simulink model "hware_long"  (R2012b)
settings: Solver=ode45  StartTime=0.0  StopTime=1500  RelTol=1e-3
libraries: xbsIndex_r4 x265, xps_library x7, casper_library_misc x2, casper_library_delays x2, casper_library_reorder x1
(part 2 of 4)

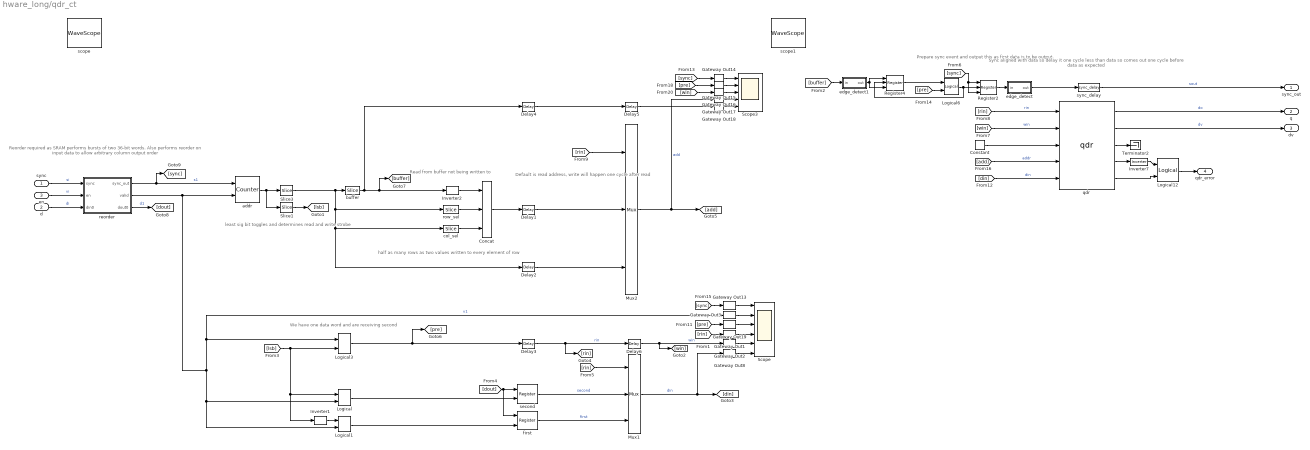
== system hware_long/qdr_ct ==
  note: Reorder required as SRAM performs
      | bursts of two 36-bit words.
      | Also performs reorder on input
      | data to allow arbitrary column
      | output order
  note: Prepare sync event and output
      | this as first data is to be output.
  note: Sync aligned with data so
      | delay it one cycle less
      | than data so comes out one
      | cycle before data as
      | expected
  note: least sig bit toggles
      | and determines read
      | and write strobe
  note: We have one data word
      | and are receiving second
  note: Default is read address,
      | write will happen one
      | cycle after read
  note: Read from buffer
      | not being
      | written to
  note: half as many rows
      | as two values
      | written to every
      | element of row
  sync : Inport
  d : Inport  Port=2
  en : Inport  Port=3
  Concat : xbsIndex_r4/Concat  num_inputs=3  dbl_ovrd=off  block_type=concat
      settings: block_version=10.1.3
  Constant : xbsIndex_r4/Constant  const=15  gui_display_data_type=Fixed-point  arith_type=Unsigned  n_bits=4  bin_pt=0  preci_type=Single  exp_width=8  frac_width=24  explicit_period=on  period=1  equ=P=C  opselect=C  inp2=PCIN>>17  opr=+  inp1=P  carry=CIN  dbl_ovrd=off  block_type=constant
  Delay{1..6} (6 alike) : xbsIndex_r4/Delay  rst=off  infoeditControl=Selection of Reset will increase slice count due to use of real FFs and instead of SRLs  en=off  latency=1  dbl_ovrd=off  reg_retiming=off  block_type=delay
      settings: block_version=11.4
  Gateway Out{1..3,8,13..19} (11 alike) : xbsIndex_r4/Gateway Out  inherit_from_input=off  hdl_port=off  timing_constraint=None  locs_specified=off  LOCs={}  UseAsDAC=off  DACChannel='1'  block_type=gatewayout
      settings: infoedit="Gateway out block.  Converts Xilinx fixed point inputs into ouputs of type Simulink integer, double, or fixed point.<br><br>Hardware notes:  In hardware these blocks become top level output ports or are discarded, depending on how they are configured."  block_version=11.4
  Inverter1 : xbsIndex_r4/Inverter  en=off  latency=0  dbl_ovrd=off  block_type=inv
  Inverter2 : xbsIndex_r4/Inverter  en=off  latency=0  dbl_ovrd=off  block_type=inv
  Inverter7 : xbsIndex_r4/Inverter  en=off  latency=0  dbl_ovrd=off  block_type=inv
      settings: block_version=11.4
  Logical{,1,3,6} (4 alike) : xbsIndex_r4/Logical  logical_function=AND  inputs=2  en=off  latency=0  precision=Full  arith_type=Unsigned  n_bits=16  bin_pt=0  align_bp=on  dbl_ovrd=off  block_type=logical
      settings: block_version=11.4
  Logical12 : xbsIndex_r4/Logical  logical_function=OR  inputs=2  en=off  latency=1  precision=Full  arith_type=Unsigned  n_bits=8  bin_pt=2  align_bp=on  dbl_ovrd=off  block_type=logical
      settings: xl_area=[0, 0, 0, 0, 0, 0, 0]
  Mux1 : xbsIndex_r4/Mux  inputs=2  en=off  latency=1  precision=Full  arith_type=Unsigned  n_bits=16  bin_pt=14  quantization=Truncate  overflow=Wrap  dbl_ovrd=off  block_type=mux
      settings: block_version=11.4
  Mux2 : xbsIndex_r4/Mux  inputs=2  en=off  latency=1  precision=Full  arith_type=Unsigned  n_bits=16  bin_pt=14  quantization=Truncate  overflow=Wrap  dbl_ovrd=off  block_type=mux
      settings: block_version=11.4
  Register2 : xbsIndex_r4/Register  init=0  rst=on  en=on  dbl_ovrd=off  block_type=register
      settings: block_version=11.4
  Register4 : xbsIndex_r4/Register  init=0  rst=on  en=on  dbl_ovrd=off  block_type=register
      settings: block_version=11.4
  Scope : Scope  NumInputPorts=6
      settings: YMin=0~0~0~0~0~0  YMax=1~1~1~1~1~15
  Scope3 : Scope  NumInputPorts=5
      settings: TimeRange=27.56125882301808  YMin=0~0~0~0~0  YMax=1~1~600~15~1  SaveName=ScopeData4
  Slice1 : xbsIndex_r4/Slice  nbits=1  boolean_output=on  mode=Lower Bit Location + Width  bit1=0  base1=MSB of Input  bit0=0  base0=LSB of Input  dbl_ovrd=off  block_type=slice
      settings: block_version=10.1.3
  Slice3 : xbsIndex_r4/Slice  nbits=(idepth + odepth + 1) - 1  boolean_output=off  mode=Upper Bit Location + Width  bit1=0  base1=MSB of Input  bit0=0  base0=LSB of Input  dbl_ovrd=off  block_type=slice
      settings: block_version=10.1.3
  Terminator2 : Terminator
  addr : xbsIndex_r4/Counter  cnt_type=Free Running  cnt_to=Inf  operation=Up  start_count=0  cnt_by_val=1  arith_type=Unsigned  n_bits=(idepth + odepth + 1)  bin_pt=0  load_pin=off  rst=on  en=on  explicit_period=on  period=1  dbl_ovrd=off  use_behavioral_HDL=off  implementation=Fabric  use_rpm=off  block_type=counter
  buffer : xbsIndex_r4/Slice  nbits=1  boolean_output=on  mode=Upper Bit Location + Width  bit1=0  base1=MSB of Input  bit0=0  base0=LSB of Input  dbl_ovrd=off  block_type=slice
      settings: block_version=10.1.3
  col_sel : xbsIndex_r4/Slice  nbits=idepth  boolean_output=off  mode=Lower Bit Location + Width  bit1=0  base1=MSB of Input  bit0=odepth-1  base0=LSB of Input  dbl_ovrd=off  block_type=slice
      settings: block_version=10.1.3
  edge_detect : Subsystem  AncestorBlock=casper_library_misc/edge_detect  mask(edge_detect){edge=Falling, polarity=Active High, x_in=[0 0.08 0.08 0.16 0.16 0.24 0.24 0.32 0.32 0.4], y_in=[1  1 -1 -1 -1 -1 -1 -1 -1 -1], x_out=[0.6 0.68 0.68 0.76 0.76 0.84 0.84 0.92 0.92 1], y_out=[-1 -1  1  1 -1 -1 -1 -1 -1 -1]}
      mask prompts: edge "Edge Type"; polarity "Output Polarity"; x_in "Input X Positions"; y_in "Input Y Positions"; x_out "Output X Positions"; y_out "Output Y Positions"
      mask help: Output is active for one-cycle after each edge of the specified type (i.e. rising, falling or both).
      mask init:
      | edge_detect_init(gcb,...
      |     'edge',edge,...
      |     'polarity',polarity,...
      |     'x_in',x_in,...
      |     'x_out',x_out,...
      |     'y_in',y_in,...
      |     'y_out',y_out);
      | 
      | x_in_num=str2num(getfield(getfield(get_param(gcb,'UserData'),'parameters'),'x_in'));
      | x_out_num=str2num(getfield(getfield(get_param(gcb,'UserData'),'parameters'),'x_out'));
      | y_in_num=str2num(getfield(getfield(get_param(gcb,'UserData'),'parameters'),'y_in'));
      | y_out_num=str2num(getfield(getfield(get_param(gcb,'UserData'),'parameters'),'y_out'));
      settings: AttributesFormatString=|
      | falling edges
      | active high
      mask Help: Output is active for one-cycle after each edge of the specified type (i.e. rising, falling, or both).  Latency is zero.
      mask TypeOptions edge: Rising | Falling | Both
      mask TypeOptions polarity: Active High | Active Low
      mask Display:
      | plot(x_in_num,0.5+y_in_num*0.2);
      | plot(x_out_num,0.5+y_out_num*0.2);
  edge_detect1 : Subsystem  AncestorBlock=casper_library_misc/edge_detect  mask(edge_detect){edge=Rising, polarity=Active High, x_in=[0 0.08 0.08 0.16 0.16 0.24 0.24 0.32 0.32 0.4], y_in=[-1 -1  1  1  1  1  1  1  1  1], x_out=[0.6 0.68 0.68 0.76 0.76 0.84 0.84 0.92 0.92 1], y_out=[-1 -1  1  1 -1 -1 -1 -1 -1 -1]}
      mask prompts: edge "Edge Type"; polarity "Output Polarity"; x_in "Input X Positions"; y_in "Input Y Positions"; x_out "Output X Positions"; y_out "Output Y Positions"
      mask help: Output is active for one-cycle after each edge of the specified type (i.e. rising, falling or both).
      mask init: same as hware_long/qdr_ct/edge_detect
      settings: AttributesFormatString=|
      | rising edges
      | active high
      mask Help: Output is active for one-cycle after each edge of the specified type (i.e. rising, falling, or both).  Latency is zero.
      mask TypeOptions edge: Rising | Falling | Both
      mask TypeOptions polarity: Active High | Active Low
      mask Display:
      | plot(x_in_num,0.5+y_in_num*0.2);
      | plot(x_out_num,0.5+y_out_num*0.2);
  first : xbsIndex_r4/Register  init=0  rst=off  en=on  dbl_ovrd=off  block_type=register
      settings: block_version=11.4
  qdr : xps_library/qdr  Tag=xps:qdr  which_qdr=qdr0  qdr_awidth=20  use_sniffer=off
  reorder : Subsystem  AncestorBlock=casper_library_reorder/reorder  mask(reorder){map=[0   65536       1   65537       2   65538       3   65539       4   65540       5   65541       6   65542       7   65543       8   65544       9   65545      10   65546      11   65547      12   65548      13   65549      14   65550      15   65551      16   65552      17   65553      18   65554      19   65555      20   65556      21   65557      22   65558      23   65559      24   65560      25   65561      26   65562      27   65563      28   65564      29   65565      30   65566      31   65567      32   65568      33   65569      34   65570      35   65571      36   65572      37   65573      38   65574      39   65575      40   65576      41   65577      42   65578      43   65579      44   65580      45   65581      46   65582      47   65583      48   65584      49   65585      50   65586      51   65587      52   65588      53   65589      54   65590      55   65591      56   65592      57   65593      58   65594      59   65595      60   65596      61   65597      62   65598      63   65599      64   65600      65   65601      66   65602      67   65603      68   65604      69   65605      70   65606      71   65607      72   65608      73   65609      74   65610      75   65611      76   65612      77   65613      78   65614      79   65615      80   65616      81   65617      82   65618      83   65619      84   65620      85   65621      86   65622      87   65623      88   65624      89   65625      90   65626      91   65627      92   65628      93   65629      94   65630      95   65631      96   65632      97   65633      98   65634      99   65635     100   65636     101   65637     102   65638     103   65639     104   65640     105   65641     106   65642     107   65643     108   65644     109   65645     110   65646     111   65647     112   65648     113   65649     114   65650     115   65651     116   65652     117   65653     118   65654     119   65655     120   65656     121   65657     122   65658     123   65659     124   65660     125   65661     126   65662     127   65663     128   65664     129   65665     130   65666     131   65667     132   65668     133   65669     134   65670     135   65671     136   65672     137   65673     138   65674     139   65675     140   65676     141   65677     142   65678     143   65679     144   65680     145   65681     146   65682     147   65683     148   65684     149   65685     150   65686     151   65687     152   65688     153   65689     154   65690     155   65691     156   65692     157   65693     158   65694     159   65695     160   65696     161   65697     162   65698     163   65699     164   65700     165   65701     166   65702     167   65703     168   65704     169   65705     170   65706     171   65707     172   65708     173   65709     174   65710     175   65711     176   65712     177   65713     178   65714     179   65715     180   65716     181   65717     182   65718     183   65719     184   65720     185   65721     186   65722     187   65723     188   65724     189   65725     190   65726     191   65727     192   65728     193   65729     194   65730     195   65731     196   65732     197   65733     198   65734     199   65735     200   65736     201   65737     202   65738     203   65739     204   65740     205   65741     206   65742     207   65743     208   65744     209   65745     210   65746     211   65747     212   65748     213   65749     214   65750     215   65751     216   65752     217   65753     218   65754     219   65755     220   65756     221   65757     222   65758     223   65759     224   65760     225   65761     226   65762     227   65763     228   65764     229   65765     230   65766     231   65767     232   65768     233   65769     234   65770     235   65771     236   65772     237   65773     238   65774     239   65775     240   65776     241   65777     242   65778     243   65779     244   65780     245   65781     246   65782     247   65783     248   65784     249   65785 ...(+1044572 chars)], n_inputs=1, bram_latency=1, map_latency=1, double_buffer=1, bram_map=on}
      mask prompts: map "Output Order:"; n_inputs "Number of inputs"; bram_latency "BRAM Latency"; map_latency "Map Latency"; double_buffer "Double Buffer"; bram_map "Use BlockRAM for Map"
      mask init:
      | reorder_init(gcb, ...
      |     'map', map, ...
      |     'n_inputs', n_inputs, ...
      |     'bram_latency', bram_latency, ...
      |     'map_latency', map_latency, ...
      |     'double_buffer', double_buffer, ...
      |     'bram_map', bram_map);
      settings: AttributesFormatString=order=2
      mask Help: eval('xlWeb(''http://casper.berkeley.edu/wiki/Reorder'')')
  row_sel : xbsIndex_r4/Slice  nbits=odepth-1  boolean_output=off  mode=Lower Bit Location + Width  bit1=0  base1=MSB of Input  bit0=0  base0=LSB of Input  dbl_ovrd=off  block_type=slice
      settings: block_version=10.1.3
  scope : xbsIndex_r4/WaveScope  block_type=wavescope
      settings: block_version=11.4
  scope1 : xbsIndex_r4/WaveScope  block_type=wavescope
      settings: block_version=11.4
  second : xbsIndex_r4/Register  init=0  rst=off  en=on  dbl_ovrd=off  block_type=register
      settings: block_version=11.4
  sync_delay : casper_library_delays/sync_delay  DelayLen=10-1
  sync_out : Outport
  q : Outport  Port=2
  dv : Outport  Port=3
  qdr_error : Outport  Port=4
  wires:
  sync/1 -> reorder/1(sync)  "si"
  en/1 -> reorder/2(en)  "vi"
  [rin] -> qdr/1  "rin"
  [win] -> qdr/2  "win"
  Constant/1 -> qdr/3
  [add] -> qdr/4  "addr"
  qdr/5 -> Logical12/2
  qdr/4 -> Inverter7/1
  qdr/3 -> Terminator2/1
  addr/1 -> Slice1/1, Slice3/1
  Logical/1 -> second/2
  Logical1/1 -> first/2
  [rin] -> Mux1/1
  Mux1/1 -> [din], Gateway Out8/1  "din"
  [din] -> qdr/5  "din"
  buffer/1 -> [buffer], Inverter2/1, Delay4/1
  [sync] -> Register2/1, Register2/3
  Register4/1 -> Logical6/1
  [pre] -> Logical6/2
  Logical6/1 -> Register2/2, Register4/2
  Register2/1 -> edge_detect/1(in)
  edge_detect/1(out) -> sync_delay/1
  row_sel/1 -> Concat/2
  [rin] -> Mux2/1
  Concat/1 -> Delay1/1
  Inverter2/1 -> Concat/1
  [sync] -> Gateway Out13/1
  Delay3/1 -> [rin], Delay6/1  "rin"
  [buffer] -> edge_detect1/1(in)
  edge_detect1/1(out) -> Register4/1, Register4/3
  col_sel/1 -> Concat/3
  second/1 -> Mux1/2  "second"
  first/1 -> Mux1/3  "first"
  Delay6/1 -> Gateway Out2/1, [win]  "win"
  [sync] -> Gateway Out14/1
  [pre] -> Gateway Out15/1
  [win] -> Gateway Out16/1
  Gateway Out14/1 -> Scope3/1
  Gateway Out15/1 -> Scope3/2
  Gateway Out16/1 -> Scope3/3
  Gateway Out17/1 -> Scope3/4
  Gateway Out18/1 -> Scope3/5
  Logical3/1 -> Delay3/1, [pre]
  [pre] -> Gateway Out19/1
  Gateway Out13/1 -> Scope/1
  Gateway Out3/1 -> Scope/2
  Gateway Out19/1 -> Scope/3
  Gateway Out1/1 -> Scope/4
  Gateway Out2/1 -> Scope/5
  Gateway Out8/1 -> Scope/6
  Inverter1/1 -> Logical1/1
  [rin] -> Gateway Out1/1
  Slice3/1 -> buffer/1, row_sel/1, col_sel/1, Delay2/1
  Slice1/1 -> [lsb]
  [lsb] -> Logical3/2, Inverter1/1, Logical/1
  Mux2/1 -> [add], Gateway Out17/1  "add"
  Delay1/1 -> Mux2/2
  Delay2/1 -> Mux2/3
  Delay4/1 -> Delay5/1
  Delay5/1 -> Gateway Out18/1
  reorder/2(valid) -> addr/2, Logical/2, Logical1/2, Gateway Out3/1, Logical3/1  "v1"
  d/1 -> reorder/3(din0)  "di"
  reorder/3(dout0) -> [dout]  "d1"
  [dout] -> second/1, first/1
  reorder/1(sync_out) -> [sync], addr/1  "s1"
  Inverter7/1 -> Logical12/1
  Logical12/1 -> qdr_error/1
  sync_delay/1 -> sync_out/1  "sout"
  qdr/1 -> q/1  "do"
  qdr/2 -> dv/1  "dv"
